simulink model "b29"  (R2017b)
settings: Solver=VariableStepAuto  StartTime=1  StopTime=30  RelTol=1e-3
settings Model: Creator=messi  LastModifiedBy=messi

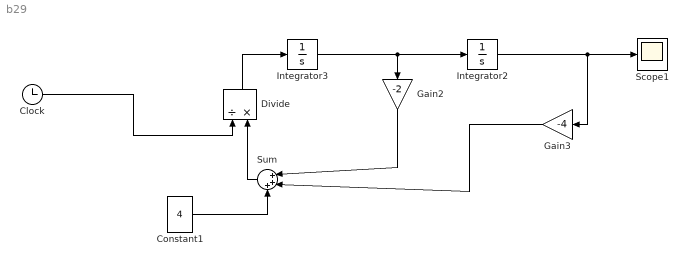
== system b29 ==
  Clock : Clock
  Constant1 : Constant  Value=4
  Divide : Product  Inputs=/*
  Gain2 : Gain  Gain=-2
  Gain3 : Gain  Gain=-4
  Integrator2 : Integrator  InitialCondition=1
  Integrator3 : Integrator  InitialCondition=1
  Scope1 : Scope
  Sum : Sum  Inputs=|+++
  wires:
  Integrator3/1 -> Gain2/1, Integrator2/1
  Integrator2/1 -> Scope1/1, Gain3/1
  Gain2/1 -> Sum/1
  Gain3/1 -> Sum/2
  Constant1/1 -> Sum/3
  Divide/1 -> Integrator3/1
  Clock/1 -> Divide/1
  Sum/1 -> Divide/2
